simulink model "rules"  (R2020b)
settings: Solver=VariableStepAuto  StartTime=0.0  StopTime=10.0  RelTol=1e-3
settings Model: Creator=xinbo  LastModifiedBy=xinbo

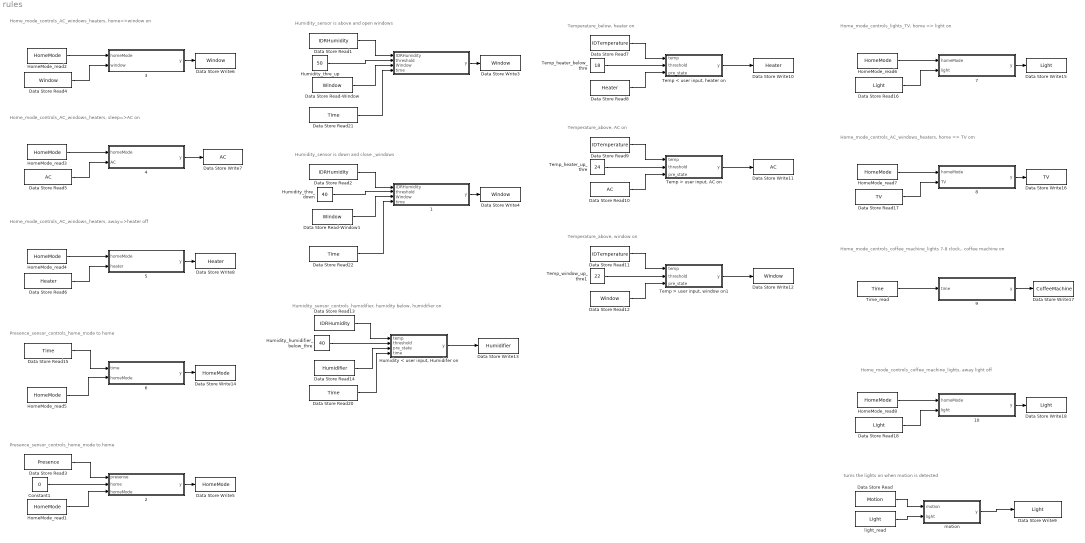
== system rules ==
  note: Humidity_sensor_controls_humidifier, humidity below, humidifier on
  note: Presence_sensor_controls_home_mode to home
  note: Home_mode_controls_AC_windows_heaters, home => TV om
  note: Home_mode_controls_coffee_machine_lights 7-8 clock,. coffee machine on
  note: Home_mode_controls_coffee_machine_lights, away light off
  note: Home_mode_controls_lights_TV, home => light on
  note: Temperature_above, window on
  note: Humidity_sensor is down and close _windows
  note: Presence_sensor_controls_home_mode to home
  note: Humidity_sensor is above and open windows
  note: turns the lights on when motion is detected
  note: Home_mode_controls_AC_windows_heaters, sleep=>AC on
  note: Home_mode_controls_AC_windows_heaters, home=>window on
  note: Home_mode_controls_AC_windows_heaters, away=>heater off
  note: Temperature_below, heater on
  note: Temperature_above, AC on
  " " : MATLAB Function  TreatAsAtomicUnit=on
  " 1" : MATLAB Function  TreatAsAtomicUnit=on
  " 10" : MATLAB Function  TreatAsAtomicUnit=on
  " 2" : MATLAB Function  TreatAsAtomicUnit=on
  " 3" : MATLAB Function  TreatAsAtomicUnit=on
  " 4" : MATLAB Function  TreatAsAtomicUnit=on
  " 5" : MATLAB Function  TreatAsAtomicUnit=on
  " 6" : MATLAB Function  TreatAsAtomicUnit=on
  " 7" : MATLAB Function  TreatAsAtomicUnit=on
  " 8" : MATLAB Function  TreatAsAtomicUnit=on
  " 9" : MATLAB Function  TreatAsAtomicUnit=on
  Constant1 : Constant  Value=0
  Data Store Read : DataStoreRead  DataStoreName=Motion
  Data Store Read1 : DataStoreRead  DataStoreName=IDRHumidity
  Data Store Read10 : DataStoreRead  DataStoreName=AC
  Data Store Read11 : DataStoreRead  DataStoreName=IDTemperature
  Data Store Read12 : DataStoreRead  DataStoreName=Window
  Data Store Read13 : DataStoreRead  DataStoreName=IDRHumidity
  Data Store Read14 : DataStoreRead  DataStoreName=Humidifier
  Data Store Read{15,20..22} (4 alike) : DataStoreRead  DataStoreName=Time
  Data Store Read16 : DataStoreRead  DataStoreName=Light
  Data Store Read17 : DataStoreRead  DataStoreName=TV
  Data Store Read18 : DataStoreRead  DataStoreName=Light
  Data Store Read2 : DataStoreRead  DataStoreName=IDRHumidity
  Data Store Read3 : DataStoreRead  DataStoreName=Presence
  Data Store Read4 : DataStoreRead  DataStoreName=Window
  Data Store Read5 : DataStoreRead  DataStoreName=AC
  Data Store Read6 : DataStoreRead  DataStoreName=Heater
  Data Store Read7 : DataStoreRead  DataStoreName=IDTemperature
  Data Store Read8 : DataStoreRead  DataStoreName=Heater
  Data Store Read9 : DataStoreRead  DataStoreName=IDTemperature
  Data Store Write10 : DataStoreWrite  DataStoreName=Heater
  Data Store Write11 : DataStoreWrite  DataStoreName=AC
  Data Store Write{3..4,6,12} (4 alike) : DataStoreWrite  DataStoreName=Window
  Data Store Write13 : DataStoreWrite  DataStoreName=Humidifier
  Data Store Write14 : DataStoreWrite  DataStoreName=HomeMode
  Data Store Write15 : DataStoreWrite  DataStoreName=Light
  Data Store Write16 : DataStoreWrite  DataStoreName=TV
  Data Store Write17 : DataStoreWrite  DataStoreName=CoffeeMachine
  Data Store Write18 : DataStoreWrite  DataStoreName=Light
  Data Store Write5 : DataStoreWrite  DataStoreName=HomeMode
  Data Store Write7 : DataStoreWrite  DataStoreName=AC
  Data Store Write8 : DataStoreWrite  DataStoreName=Heater
  Data Store Write9 : DataStoreWrite  DataStoreName=Light
  Data Store Read-Window : DataStoreRead  DataStoreName=Window
  Data Store Read-Window1 : DataStoreRead  DataStoreName=Window
  HomeMode_read{1..8} (8 alike) : DataStoreRead  DataStoreName=HomeMode
  "Humidity < user input, Humidifer on" : MATLAB Function  TreatAsAtomicUnit=on
  Humidity_humidifier_below_thre : Constant  Value=40
  Humidity_thre_down : Constant  Value=40
  Humidity_thre_up : Constant  Value=50
  "Temp < user input, heater on" : MATLAB Function  TreatAsAtomicUnit=on
  "Temp > user input, AC on" : MATLAB Function  TreatAsAtomicUnit=on
  "Temp > user input, window on1" : MATLAB Function  TreatAsAtomicUnit=on
  Temp_heater_below_thre : Constant  Value=18
  Temp_heater_up_thre : Constant  Value=24
  Temp_window_up_thre1 : Constant  Value=22
  Time_read : DataStoreRead  DataStoreName=Time
  light_read : DataStoreRead  DataStoreName=Light  SampleTime=1
  motion : MATLAB Function  TreatAsAtomicUnit=on
  wires:
  " 5"/1(y) -> Data Store Write8/1
  Data Store Read7/1 -> "Temp < user input, heater on"/1(temp)
  HomeMode_read5/1 -> " 6"/2(homeMode)
  HomeMode_read8/1 -> " 10"/1(homeMode)
  Data Store Read6/1 -> " 5"/2(heater)
  Data Store Read10/1 -> "Temp > user input, AC on"/3(pre_state)
  HomeMode_read4/1 -> " 5"/1(homeMode)
  HomeMode_read2/1 -> " 3"/1(homeMode)
  Data Store Read14/1 -> "Humidity < user input, Humidifer on"/3(pre_state)
  Time_read/1 -> " 9"/1(time)
  Data Store Read3/1 -> " 2"/1(presense)
  Data Store Read16/1 -> " 7"/2(light)
  Data Store Read4/1 -> " 3"/2(window)
  Temp_window_up_thre1/1 -> "Temp > user input, window on1"/2(threshold)
  light_read/1 -> motion/2(light)
  " 10"/1(y) -> Data Store Write18/1
  Data Store Read8/1 -> "Temp < user input, heater on"/3(pre_state)
  " 7"/1(y) -> Data Store Write15/1
  HomeMode_read3/1 -> " 4"/1(homeMode)
  Data Store Read17/1 -> " 8"/2(TV)
  " "/1(y) -> Data Store Write3/1
  "Humidity < user input, Humidifer on"/1(y) -> Data Store Write13/1
  Data Store Read18/1 -> " 10"/2(light)
  Data Store Read-Window/1 -> " "/3(Window)
  " 2"/1(y) -> Data Store Write5/1
  Temp_heater_up_thre/1 -> "Temp > user input, AC on"/2(threshold)
  " 9"/1(y) -> Data Store Write17/1
  Temp_heater_below_thre/1 -> "Temp < user input, heater on"/2(threshold)
  HomeMode_read7/1 -> " 8"/1(homeMode)
  Data Store Read15/1 -> " 6"/1(time)
  " 6"/1(y) -> Data Store Write14/1
  Data Store Read21/1 -> " "/4(time)
  Data Store Read5/1 -> " 4"/2(AC)
  Data Store Read9/1 -> "Temp > user input, AC on"/1(temp)
  Data Store Read11/1 -> "Temp > user input, window on1"/1(temp)
  Data Store Read22/1 -> " 1"/4(time)
  Constant1/1 -> " 2"/2(home)
  " 8"/1(y) -> Data Store Write16/1
  Data Store Read/1 -> motion/1(motion)
  motion/1(y) -> Data Store Write9/1
  Data Store Read1/1 -> " "/1(IDRHumidity)
  HomeMode_read1/1 -> " 2"/3(homeMode)
  Data Store Read-Window1/1 -> " 1"/3(Window)
  "Temp > user input, AC on"/1(y) -> Data Store Write11/1
  Humidity_thre_down/1 -> " 1"/2(threshold)
  Humidity_thre_up/1 -> " "/2(threshold)
  " 3"/1(y) -> Data Store Write6/1
  Data Store Read2/1 -> " 1"/1(IDRHumidity)
  Data Store Read20/1 -> "Humidity < user input, Humidifer on"/4(time)
  " 4"/1(y) -> Data Store Write7/1
  " 1"/1(y) -> Data Store Write4/1
  "Temp < user input, heater on"/1(y) -> Data Store Write10/1
  Data Store Read12/1 -> "Temp > user input, window on1"/3(pre_state)
  "Temp > user input, window on1"/1(y) -> Data Store Write12/1
  HomeMode_read6/1 -> " 7"/1(homeMode)
  Data Store Read13/1 -> "Humidity < user input, Humidifer on"/1(temp)
  Humidity_humidifier_below_thre/1 -> "Humidity < user input, Humidifer on"/2(threshold)

== matlab function rules/Humidity < user input, Humidifer on ==
  data: temp input; y output; threshold input; pre_state input; time input
function y = ST11(temp, threshold, pre_state, time)

if(temp < threshold && time > 0)
    y = 1;
else
    y = pre_state;
end

== matlab function rules/ 6 ==
  data: time input; y output; homeMode input
function y = ST11(time, homeMode)

if(time > 18 && time <23)
    y = 0;
elseif (time >23 || time < 6)
    y = 1;
elseif (time > 8 && time < 18)
    y = 2;
else
    y = homeMode;
end

== matlab function rules/ 7 ==
  data: homeMode input; light input; y output
function y = ST11(homeMode, light)

if(homeMode == 0)
    y = 1;
else
    y = light;
end

== matlab function rules/ 8 ==
  data: homeMode input; TV input; y output
function y = ST11(homeMode, TV)

if(homeMode == 1)
    y = 1;
else
    y = TV;
end

== matlab function rules/  ==
  data: IDRHumidity input; y output; threshold input; Window input; time input
function y = ST1(IDRHumidity, threshold, Window, time)

if(IDRHumidity > threshold && time > 0)
    y = 1;
else
    y = Window;
end

== matlab function rules/ 10 ==
  data: homeMode input; light input; y output
function y = ST11(homeMode, light)

if(homeMode == 2)
    y = 0;
else
    y = light;
end

== matlab function rules/ 9 ==
  data: time input; y output
function y = ST11(time)

if(time > 7 && time < 8)
    y = 1;
else
    y = 0;
end

== matlab function rules/ 1 ==
  data: IDRHumidity input; y output; threshold input; Window input; time input
function y = ST1(IDRHumidity, threshold, Window, time)

if(IDRHumidity < threshold && time > 0)
    y = 0;
else
    y = Window;
end

== matlab function rules/ 2 ==
  data: presense input; y output; home input; homeMode input
function y = ST11(presense, home, homeMode)

if(presense > 0)
    y = home;
else
    y = homeMode;
end

== matlab function rules/ 3 ==
  data: homeMode input; window input; y output
function y = ST11(homeMode, window)

if(homeMode == 0)
    y = 1;
else
    y = window;
end

== matlab function rules/ 4 ==
  data: homeMode input; AC input; y output
function y = ST11(homeMode, AC)

if(homeMode == 1)
    y = 1;
else
    y = AC;
end

== matlab function rules/ 5 ==
  data: homeMode input; heater input; y output
function y = ST11(homeMode, heater)

if(homeMode == 2)
    y = 0;
else
    y = heater;
end

== matlab function rules/motion ==
  data: motion input; y output; light input
function y= motionMode(motion,light)

if(motion == 1)
    y = 1;
else
    y = light;
end

== matlab function rules/Temp > user input, AC on ==
  data: temp input; y output; threshold input; pre_state input
function y = ST11(temp, threshold, pre_state)

if(temp > threshold)
    y = 1;
else
    y = pre_state;
end

== matlab function rules/Temp < user input, heater on ==
  data: temp input; y output; threshold input; pre_state input
function y = ST11(temp, threshold, pre_state)

if(temp < threshold)
    y = 1;
else
    y = pre_state;
end

== matlab function rules/Temp > user input, window on1 ==
  data: temp input; y output; threshold input; pre_state input
function y = ST11(temp, threshold, pre_state)

if(temp > threshold)
    y = 1;
else
    y = pre_state;
end
